simulink library "INT_RmtAPP_Plaus12"  (R2016b)
settings: Solver=VariableStepAuto  StartTime=0.0  StopTime=10.0  RelTol=1e-3
settings Model: Creator=bianxuyin  LastModifiedBy=bianxuyin

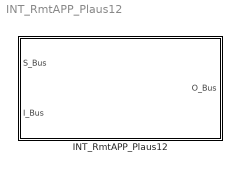
== system INT_RmtAPP_Plaus12 ==
  INT_RmtAPP_Plaus12 : Subsystem

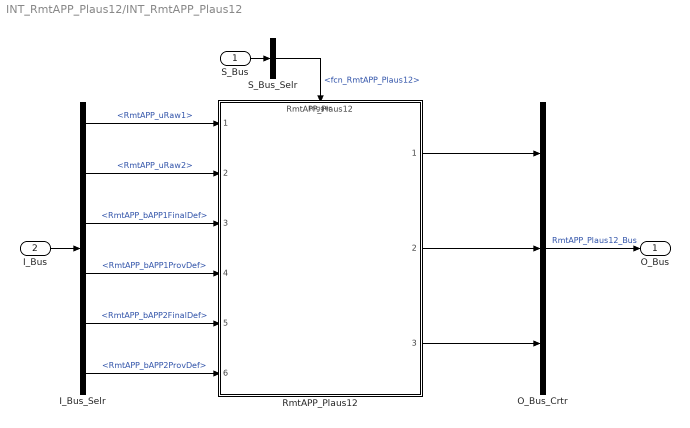
== system INT_RmtAPP_Plaus12/INT_RmtAPP_Plaus12 ==
  S_Bus : Inport
  I_Bus : Inport  Port=2
  I_Bus_Selr : BusSelector  OutputSignals=RmtAPP_uRaw1,RmtAPP_uRaw2,RmtAPP_bAPP1FinalDef,RmtAPP_bAPP1ProvDef,RmtAPP_bAPP2FinalDef,RmtAPP_bAPP2ProvDef
  O_Bus_Crtr : BusCreator  Inputs=3
  RmtAPP_Plaus12 : ModelReference  ModelNameDialog=RmtAPP_Plaus12  SimulationMode=Normal  ModelReferenceVersion=1.6  TriggerPortName=function  TriggerPortTriggerType=function-call  TriggerPortStatesWhenEnabling=held
  S_Bus_Selr : BusSelector  OutputSignals=fcn_RmtAPP_Plaus12
  O_Bus : Outport
  wires:
  S_Bus_Selr/1 -> RmtAPP_Plaus12/Trigger  "<fcn_RmtAPP_Plaus12>"
  S_Bus/1 -> S_Bus_Selr/1
  I_Bus/1 -> I_Bus_Selr/1
  I_Bus_Selr/1 -> RmtAPP_Plaus12/1  "<RmtAPP_uRaw1>"
  I_Bus_Selr/2 -> RmtAPP_Plaus12/2  "<RmtAPP_uRaw2>"
  I_Bus_Selr/3 -> RmtAPP_Plaus12/3  "<RmtAPP_bAPP1FinalDef>"
  I_Bus_Selr/4 -> RmtAPP_Plaus12/4  "<RmtAPP_bAPP1ProvDef>"
  I_Bus_Selr/5 -> RmtAPP_Plaus12/5  "<RmtAPP_bAPP2FinalDef>"
  I_Bus_Selr/6 -> RmtAPP_Plaus12/6  "<RmtAPP_bAPP2ProvDef>"
  O_Bus_Crtr/1 -> O_Bus/1  "RmtAPP_Plaus12_Bus"
  RmtAPP_Plaus12/1 -> O_Bus_Crtr/1
  RmtAPP_Plaus12/2 -> O_Bus_Crtr/2
  RmtAPP_Plaus12/3 -> O_Bus_Crtr/3
